simulink model "sovai"  (Simulink 7.5)
settings: Solver=ode45  StartTime=0.0  StopTime=150  FixedStep=1e-2  RelTol=1e-1
PostLoadFcn:
  | % Import the data from Excel for a lookup table
  | data = xlsread('MySpreadsheet','Sheet1');
  | % Row indices for lookup table
  | breakpoints1 = data(2:end,1)';
  | % Column indices for lookup table
  | breakpoints2 = data(1,2:end);
  | % Output values for lookup table
  | table_data = data(2:end,2:end);
values from neighbouring files (symbols this model uses):
  aderdin = 0.8    [InitialParameters.m]
  aderest = 0.88    [InitialParameters.m]
  cons120 = 8.79765621    [InitialParameters.m]
  cons60 = 2.81797722    [InitialParameters.m]
  cons80 = 3.91048967    [InitialParameters.m]
  consvmax = 15.01318082    [InitialParameters.m]
  efemb = [1+cos(-pi+pi*tembc/tefmax)]/2    [InitialParameters.m]
  F0 = 96.9    [InitialParameters.m]
  F2 = 0.502    [InitialParameters.m]
  g = 9.81    [InitialParameters.m]
  m = 825    [InitialParameters.m]
  M1 = 4.273    [InitialParameters.m]
  M2 = 2.238    [InitialParameters.m]
  M3 = 1.444    [InitialParameters.m]
  M4 = 1.029    [InitialParameters.m]
  M5 = 0.838    [InitialParameters.m]
  M6 = 0.838    [InitialParameters.m]
  Md = 4.067    [InitialParameters.m]
  Nfr = 0.6*m*g    (= 4855.95)    [InitialParameters.m]
  Ni = 0.94    [InitialParameters.m]
  Nmax = 6500    [InitialParameters.m]
  Nmin = 1500    [InitialParameters.m]
  Pot = [16.4 19.5 21.9 25.7 29.7 32.8 36.0 38.8 41.4 44.1 47.9 51.9 54.7 57.1 59.2 60.9 61.1 60.9 59.8 59.7 59.3]    [InitialParameters.m]
  rd = 0.274    [InitialParameters.m]
  Rot = [1500 1750 2000 2250 2500 2750 3000 3250 3500 3750 4000 4250 4500 4750 5000 5250 5500 5750 6000 6250 6500]    [InitialParameters.m]
  temb = [temb1,temb2]    [InitialParameters.m]
  teta = 0    [InitialParameters.m]
  Tor = [7.83 7.98 7.84 8.18 8.51 8.54 8.59 8.55 8.47 8.42 8.58 8.75 8.71 8.61 8.48 8.31 7.96 7.59 7.14 6.84 6.53]    [InitialParameters.m]
  Vini = 0    [InitialParameters.m]
libraries: simulink x5, dspswit3 x2
settings Model: Creator=Bruno Silva de Lima  LastModifiedBy=user
settings DebuggingCC: StrictBusMsg=Warning

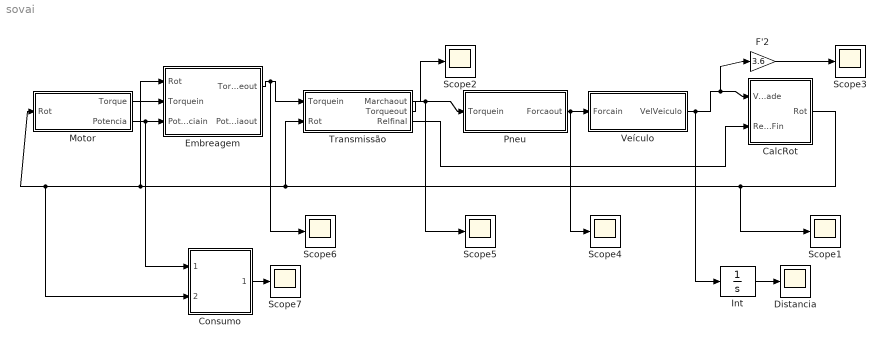
== system sovai ==
  CalcRot : Subsystem
  Consumo : Subsystem
  Distancia : Scope
      settings: SaveName=ScopeData24
  Embreagem : Subsystem  TreatAsAtomicUnit=on
  F'2 : Gain  Gain=3.6  ParameterDataType=fixdt(1, 16)  ParameterScaling=2^0  OutDataType=fixdt(1, 16)  OutScaling=2^0
  Int : Integrator  InitialCondition=Vini
  Motor : Subsystem  TreatAsAtomicUnit=on
  Pneu : Subsystem  TreatAsAtomicUnit=on
  Scope{1..7} (7 alike) : Scope
      Scope1 settings: TimeRange=150  YMin=1500  YMax=6500  MaxDataPoints=200000
      Scope2 settings: SaveName=ScopeData2
      Scope3 settings: TimeRange=0.02579854948784544  YMin=99.96457640249099  YMax=99.99862765668536  SaveName=ScopeData4
      Scope4 settings: SaveName=ScopeData3
      Scope5 settings: SaveName=ScopeData6
      Scope6 settings: SaveName=ScopeData5
      Scope7 settings: SaveName=ScopeData16
  Transmissão : Subsystem  TreatAsAtomicUnit=on
  Veículo : Subsystem  TreatAsAtomicUnit=on
  wires:
  Transmissão/2(Torqueout) -> Pneu/1(Torquein), Scope5/1
  Pneu/1(Forcaout) -> Veículo/1(Forcain), Scope4/1
  Transmissão/3(Relfinal) -> CalcRot/2(RelaçãoFin)
  CalcRot/1(Rot) -> Transmissão/2(Rot), Embreagem/1(Rot), Motor/1(Rot), Consumo/2(rotacao), Scope1/1
  Motor/1(Torque) -> Embreagem/2(Torquein)
  Motor/2(Potencia) -> Embreagem/3(Potênciain), Consumo/1(Potencia)
  Embreagem/1(Torqueout) -> Transmissão/1(Torquein), Scope6/1
  Veículo/1(VelVeiculo) -> CalcRot/1(Velocidade), F'2/1, Int/1
  Transmissão/1(Marchaout) -> Scope2/1
  Consumo/1(consumo) -> Scope7/1
  F'2/1 -> Scope3/1
  Int/1 -> Distancia/1

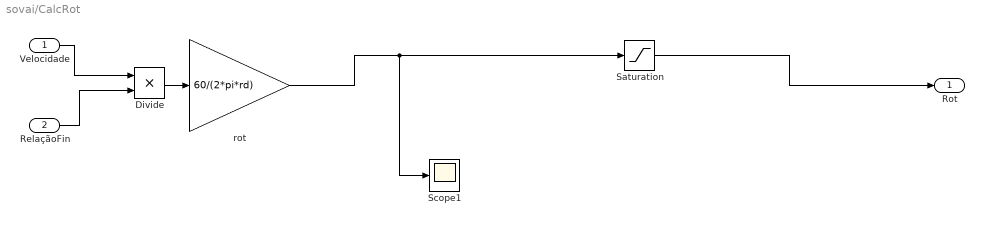
== system sovai/CalcRot ==
  Velocidade : Inport
  RelaçãoFin : Inport  Port=2
  Divide : Product  Inputs=**  OutDataType=fixdt(1, 16)  OutScaling=2^-10
  Saturation : Saturate  UpperLimit=Nmax  LowerLimit=Nmin  OutDataType=fixdt(1, 16)  OutScaling=2^0
  Scope1 : Scope
      settings: SaveName=ScopeData12
  rot : Gain  Gain=60/(2*pi*rd)  ParameterDataType=fixdt(1, 16)  ParameterScaling=2^0  OutDataType=fixdt(1, 16)  OutScaling=2^0
  Rot : Outport
  wires:
  RelaçãoFin/1 -> Divide/2
  Velocidade/1 -> Divide/1
  Divide/1 -> rot/1
  rot/1 -> Scope1/1, Saturation/1
  Saturation/1 -> Rot/1

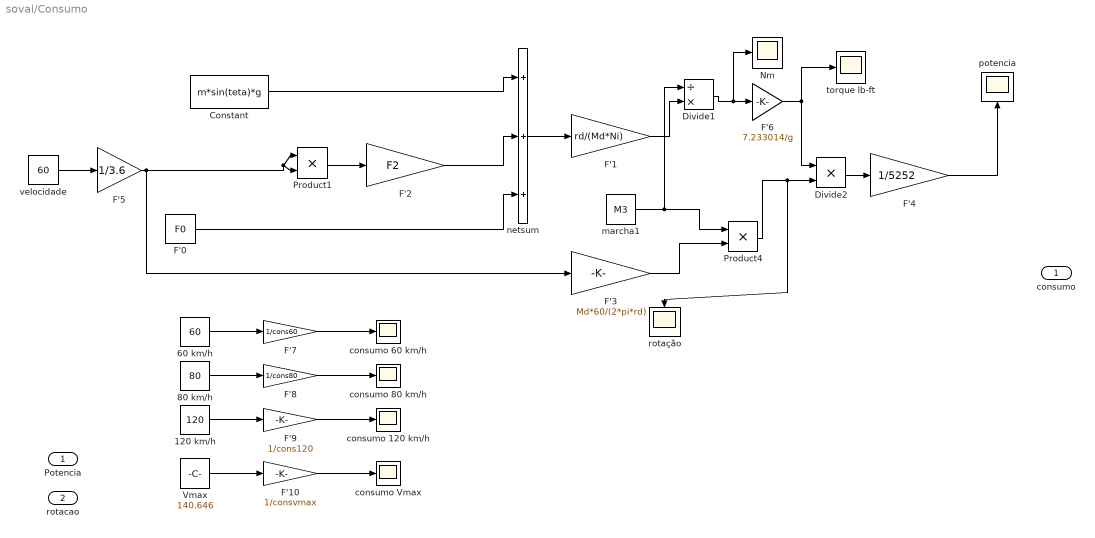
== system sovai/Consumo ==
  Potencia : Inport
  rotacao : Inport  Port=2
  120 km/h : Constant  Value=120  OutDataType=fixdt(1, 16)  OutScaling=2^0
  60 km/h : Constant  Value=60  OutDataType=fixdt(1, 16)  OutScaling=2^0
  80 km/h : Constant  Value=80  OutDataType=fixdt(1, 16)  OutScaling=2^0
  Constant : Constant  Value=m*sin(teta)*g  OutDataType=fixdt(1, 16)  OutScaling=2^0
  Divide1 : Product  Inputs=/*  OutDataType=fixdt(1, 16)  OutScaling=2^-10
  Divide2 : Product  Inputs=**  OutDataType=fixdt(1, 16)  OutScaling=2^-10
  F'0 : Constant  Value=F0  OutDataType=fixdt(1, 16)  OutScaling=2^0
  F'1 : Gain  Gain=rd/(Md*Ni)  ParameterDataType=fixdt(1, 16)  ParameterScaling=2^0  OutDataType=fixdt(1, 16)  OutScaling=2^0
  F'10 : Gain  Gain=1/consvmax  ParameterDataType=fixdt(1, 16)  ParameterScaling=2^0  OutDataType=fixdt(1, 16)  OutScaling=2^0
  F'2 : Gain  Gain=F2  ParameterDataType=fixdt(1, 16)  ParameterScaling=2^0  OutDataType=fixdt(1, 16)  OutScaling=2^0
  F'3 : Gain  Gain=Md*60/(2*pi*rd)  ParameterDataType=fixdt(1, 16)  ParameterScaling=2^0  OutDataType=fixdt(1, 16)  OutScaling=2^0
  F'4 : Gain  Gain=1/5252  ParameterDataType=fixdt(1, 16)  ParameterScaling=2^0  OutDataType=fixdt(1, 16)  OutScaling=2^0
  F'5 : Gain  Gain=1/3.6  ParameterDataType=fixdt(1, 16)  ParameterScaling=2^0  OutDataType=fixdt(1, 16)  OutScaling=2^0
  F'6 : Gain  Gain=7.233014/g  ParameterDataType=fixdt(1, 16)  ParameterScaling=2^0  OutDataType=fixdt(1, 16)  OutScaling=2^0
  F'7 : Gain  Gain=1/cons60  ParameterDataType=fixdt(1, 16)  ParameterScaling=2^0  OutDataType=fixdt(1, 16)  OutScaling=2^0
  F'8 : Gain  Gain=1/cons80  ParameterDataType=fixdt(1, 16)  ParameterScaling=2^0  OutDataType=fixdt(1, 16)  OutScaling=2^0
  F'9 : Gain  Gain=1/cons120  ParameterDataType=fixdt(1, 16)  ParameterScaling=2^0  OutDataType=fixdt(1, 16)  OutScaling=2^0
  Nm : Scope
      settings: SaveName=ScopeData20
  Product1 : Product  OutDataType=fixdt(1, 16)  OutScaling=2^0  RndMeth=Zero
  Product4 : Product  OutDataType=fixdt(1, 16)  OutScaling=2^0  RndMeth=Zero
  Vmax : Constant  Value=140.646  OutDataType=fixdt(1, 16)  OutScaling=2^0
  consumo 120 km/h : Scope
      settings: SaveName=ScopeData22
  consumo 60 km/h : Scope
  consumo 80 km/h : Scope
      settings: SaveName=ScopeData21
  consumo Vmax : Scope
      settings: SaveName=ScopeData23
  marcha1 : Constant  Value=M3  OutDataType=fixdt(1, 16)  OutScaling=2^0
  netsum : Sum  Inputs=+++  OutDataType=sfix(16)  OutScaling=2^0  SaturateOnIntegerOverflow=on  InputSameDT=on  OutDataTypeStr=Inherit: Same as first input
  potencia : Scope
      settings: SaveName=ScopeData18
  rotação : Scope
      settings: SaveName=ScopeData17
  torque lb-ft : Scope
      settings: SaveName=ScopeData19
  velocidade : Constant  Value=60  OutDataType=fixdt(1, 16)  OutScaling=2^0
  consumo : Outport
  wires:
  Constant/1 -> netsum/1
  F'2/1 -> netsum/2
  Product1/1 -> F'2/1
  F'0/1 -> netsum/3
  velocidade/1 -> F'5/1
  netsum/1 -> F'1/1
  F'1/1 -> Divide1/2
  F'3/1 -> Product4/2
  marcha1/1 -> Product4/1, Divide1/1
  Product4/1 -> rotação/1, Divide2/2
  Divide1/1 -> F'6/1, Nm/1
  Divide2/1 -> F'4/1
  F'4/1 -> potencia/1
  F'5/1 -> Product1/1, Product1/2, F'3/1
  F'6/1 -> Divide2/1, torque lb-ft/1
  60 km/h/1 -> F'7/1
  80 km/h/1 -> F'8/1
  120 km/h/1 -> F'9/1
  Vmax/1 -> F'10/1
  F'9/1 -> consumo 120 km/h/1
  F'8/1 -> consumo 80 km/h/1
  F'7/1 -> consumo 60 km/h/1
  F'10/1 -> consumo Vmax/1

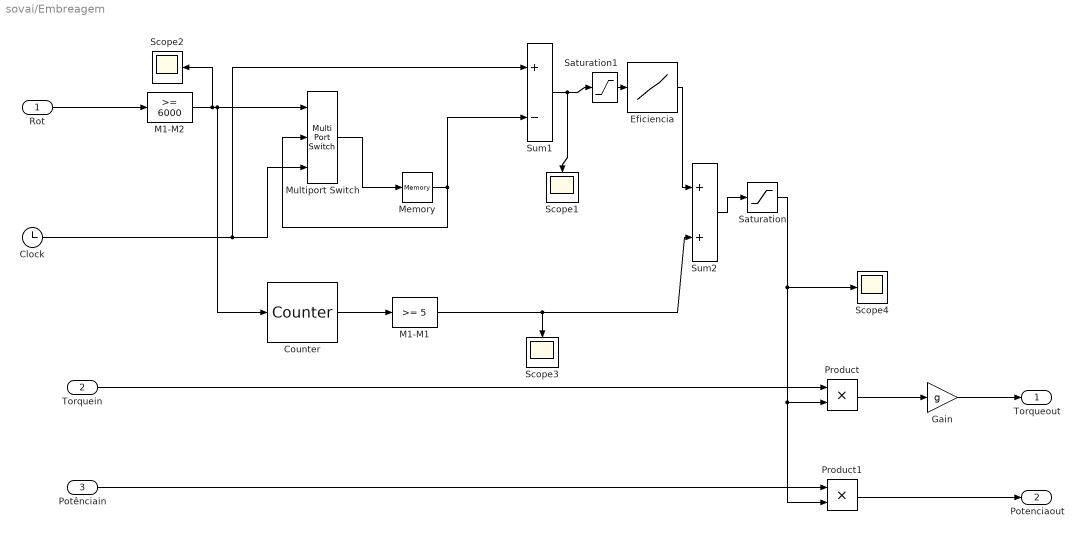
== system sovai/Embreagem ==
  Rot : Inport  OutDataType=fixdt(1, 16)  OutScaling=2^0
  Torquein : Inport  Port=2  OutDataType=fixdt(1, 16)  OutScaling=2^0
  Potênciain : Inport  Port=3  OutDataType=fixdt(1, 16)  OutScaling=2^0
  Clock : Clock
      settings: Decimation=10
  Counter : dspswit3/Counter  Direction=Up  CountEvent=Rising edge  CounterSize=User defined  MaxCount=6  InitialCount=1  Output=Count  HitValue=32  ResetInput=off  SamplesPerFrame=1  Ts=1  CntDtype=double  HitDtype=Logical
  Eficiencia : Lookup  InputValues=temb  Table=efemb  OutDataType=fixdt(1, 16)  OutScaling=2^0
  Gain : Gain  Gain=g  ParameterDataType=fixdt(1, 16)  ParameterScaling=2^0  OutDataType=fixdt(1, 16)  OutScaling=2^0
  M1-M1 : simulink/Logic and Bit Operations/Compare To Constant  SystemSampleTime=-1  relop=>=  const=5  LogicOutDataTypeMode=uint8
  M1-M2 : simulink/Logic and Bit Operations/Compare To Constant  SystemSampleTime=-1  relop=>=  const=6000  LogicOutDataTypeMode=uint8
  Memory : Memory
  Multiport Switch : MultiPortSwitch  DataPortOrder=Zero-based contiguous  Inputs=2  zeroidx=on  OutDataType=fixdt(1, 16)  OutScaling=2^0
  Product : Product  OutDataType=fixdt(1, 16)  OutScaling=2^0  RndMeth=Zero
  Product1 : Product  OutDataType=fixdt(1, 16)  OutScaling=2^0  RndMeth=Zero
  Saturation : Saturate  UpperLimit=1  LowerLimit=0  OutDataType=fixdt(1, 16)  OutScaling=2^0
  Saturation1 : Saturate  UpperLimit=1.5  LowerLimit=0  OutDataType=fixdt(1, 16)  OutScaling=2^0
  Scope{1..4} (4 alike) : Scope
      Scope1 settings: SaveName=ScopeData13
      Scope2 settings: SaveName=ScopeData14
      Scope3 settings: SaveName=ScopeData9
      Scope4 settings: SaveName=ScopeData25
  Sum1 : Sum  Inputs=+-  OutDataType=fixdt(1, 16)  OutScaling=2^0
  Sum2 : Sum  Inputs=2  OutDataType=fixdt(1, 16)  OutScaling=2^0
  Torqueout : Outport  OutDataType=fixdt(1, 16)  OutScaling=2^0
  Potenciaout : Outport  Port=2  OutDataType=fixdt(1, 16)  OutScaling=2^0
  wires:
  Product/1 -> Gain/1
  Product1/1 -> Potenciaout/1
  Torquein/1 -> Product/1
  Potênciain/1 -> Product1/1
  Rot/1 -> M1-M2/1
  Saturation/1 -> Product1/2, Product/2, Scope4/1
  Saturation1/1 -> Eficiencia/1
  Multiport Switch/1 -> Memory/1
  Memory/1 -> Sum1/2, Multiport Switch/2
  Clock/1 -> Multiport Switch/3, Sum1/1
  Sum1/1 -> Saturation1/1, Scope1/1
  Gain/1 -> Torqueout/1
  M1-M2/1 -> Scope2/1, Multiport Switch/1, Counter/1
  Counter/1 -> M1-M1/1
  M1-M1/1 -> Sum2/2, Scope3/1
  Sum2/1 -> Saturation/1
  Eficiencia/1 -> Sum2/1

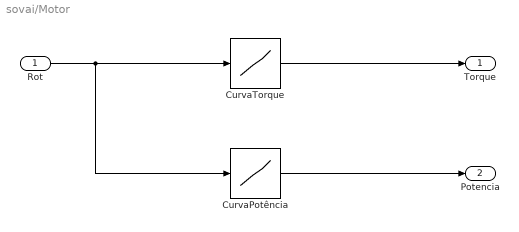
== system sovai/Motor ==
  Rot : Inport  OutDataType=fixdt(1, 16)  OutScaling=2^0
  CurvaPotência : Lookup  InputValues=Rot  Table=Pot  OutDataType=fixdt(1, 16)  OutScaling=2^0
  CurvaTorque : Lookup  InputValues=Rot  Table=Tor  OutDataType=fixdt(1, 16)  OutScaling=2^0
  Torque : Outport  OutDataType=fixdt(1, 16)  OutScaling=2^0
  Potencia : Outport  Port=2  OutDataType=fixdt(1, 16)  OutScaling=2^0
  wires:
  CurvaTorque/1 -> Torque/1
  CurvaPotência/1 -> Potencia/1
  Rot/1 -> CurvaTorque/1, CurvaPotência/1

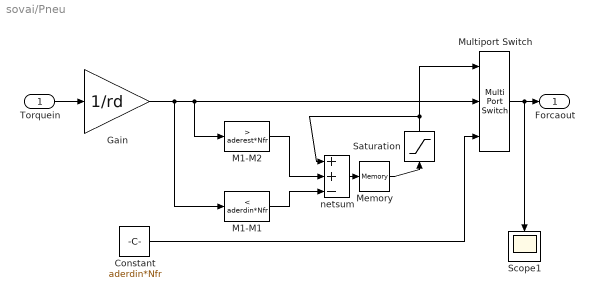
== system sovai/Pneu ==
  Torquein : Inport  OutDataType=fixdt(1, 16)  OutScaling=2^0
  Constant : Constant  Value=aderdin*Nfr  OutDataType=fixdt(1, 16)  OutScaling=2^0
  Gain : Gain  Gain=1/rd  ParameterDataType=fixdt(1, 16)  ParameterScaling=2^0  OutDataType=fixdt(1, 16)  OutScaling=2^0
  M1-M1 : simulink/Logic and Bit Operations/Compare To Constant  SystemSampleTime=-1  relop=<  const=aderdin*Nfr  LogicOutDataTypeMode=uint8
  M1-M2 : simulink/Logic and Bit Operations/Compare To Constant  SystemSampleTime=-1  relop=>  const=aderest*Nfr  LogicOutDataTypeMode=uint8
  Memory : Memory
  Multiport Switch : MultiPortSwitch  DataPortOrder=Zero-based contiguous  Inputs=2  zeroidx=on  OutDataType=fixdt(1, 16)  OutScaling=2^0
  Saturation : Saturate  UpperLimit=1  LowerLimit=0  OutDataType=fixdt(1, 16)  OutScaling=2^0
  Scope1 : Scope
      settings: SaveName=ScopeData26  MaxDataPoints=200000
  netsum : Sum  Inputs=++-  OutDataType=sfix(16)  OutScaling=2^0  SaturateOnIntegerOverflow=on  InputSameDT=on  OutDataTypeStr=Inherit: Same as first input
  Forcaout : Outport  OutDataType=fixdt(1, 16)  OutScaling=2^0
  wires:
  Torquein/1 -> Gain/1
  Multiport Switch/1 -> Forcaout/1, Scope1/1
  Constant/1 -> Multiport Switch/3
  Memory/1 -> Saturation/1
  M1-M2/1 -> netsum/2
  M1-M1/1 -> netsum/3
  netsum/1 -> Memory/1
  Saturation/1 -> Multiport Switch/1, netsum/1
  Gain/1 -> Multiport Switch/2, M1-M2/1, M1-M1/1

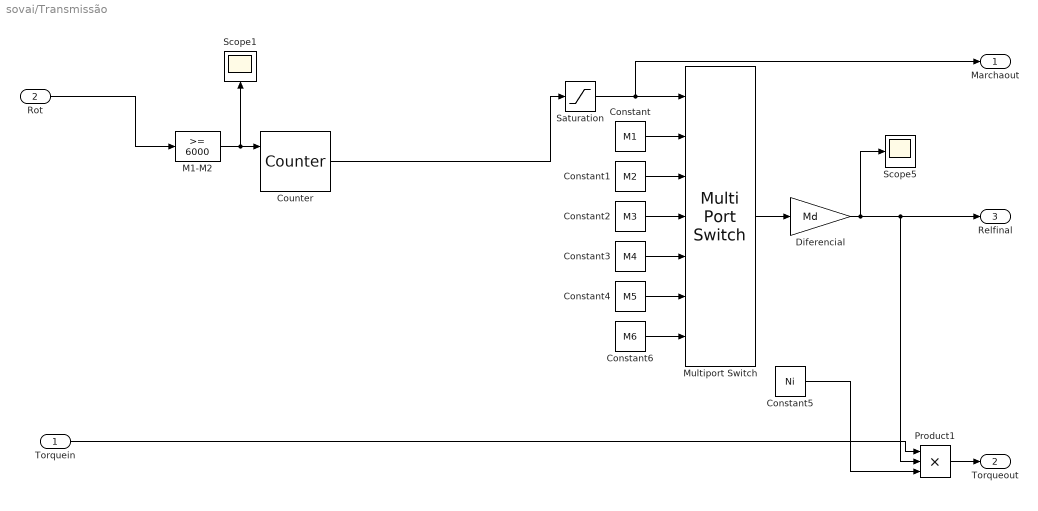
== system sovai/Transmissão ==
  Torquein : Inport  OutDataType=fixdt(1, 16)  OutScaling=2^0
  Rot : Inport  Port=2  OutDataType=fixdt(1, 16)  OutScaling=2^0
  Constant : Constant  Value=M1  OutDataType=fixdt(1, 16)  OutScaling=2^0
  Constant1 : Constant  Value=M2  OutDataType=fixdt(1, 16)  OutScaling=2^0
  Constant2 : Constant  Value=M3  OutDataType=fixdt(1, 16)  OutScaling=2^0
  Constant3 : Constant  Value=M4  OutDataType=fixdt(1, 16)  OutScaling=2^0
  Constant4 : Constant  Value=M5  OutDataType=fixdt(1, 16)  OutScaling=2^0
  Constant5 : Constant  Value=Ni  OutDataType=fixdt(1, 16)  OutScaling=2^0
  Constant6 : Constant  Value=M6  OutDataType=fixdt(1, 16)  OutScaling=2^0
  Counter : dspswit3/Counter  Direction=Up  CountEvent=Rising edge  CounterSize=User defined  MaxCount=6  InitialCount=1  Output=Count  HitValue=32  ResetInput=on  SamplesPerFrame=1  Ts=1  CntDtype=double  HitDtype=Logical
  Diferencial : Gain  Gain=Md  ParameterDataType=fixdt(1, 16)  ParameterScaling=2^0  OutDataType=fixdt(1, 16)  OutScaling=2^0
  M1-M2 : simulink/Logic and Bit Operations/Compare To Constant  SystemSampleTime=-1  relop=>=  const=6000  LogicOutDataTypeMode=uint8
  Multiport Switch : MultiPortSwitch  Inputs=6  zeroidx=off  OutDataType=fixdt(1, 16)  OutScaling=2^0
  Product1 : Product  Inputs=3  OutDataType=fixdt(1, 16)  OutScaling=2^0  RndMeth=Zero
  Saturation : Saturate  UpperLimit=4  LowerLimit=1  OutDataType=fixdt(1, 16)  OutScaling=2^0
  Scope1 : Scope
      settings: SaveName=ScopeData15
  Scope5 : Scope
      settings: SaveName=ScopeData11
  Marchaout : Outport  OutDataType=fixdt(1, 16)  OutScaling=2^0
  Torqueout : Outport  Port=2  OutDataType=fixdt(1, 16)  OutScaling=2^0
  Relfinal : Outport  Port=3  OutDataType=fixdt(1, 16)  OutScaling=2^0
  wires:
  Constant/1 -> Multiport Switch/2
  Constant1/1 -> Multiport Switch/3
  Constant2/1 -> Multiport Switch/4
  Constant3/1 -> Multiport Switch/5
  Constant4/1 -> Multiport Switch/6
  Constant6/1 -> Multiport Switch/7
  Product1/1 -> Torqueout/1
  Torquein/1 -> Product1/1
  Diferencial/1 -> Scope5/1, Product1/2, Relfinal/1
  Saturation/1 -> Multiport Switch/1, Marchaout/1
  Constant5/1 -> Product1/3
  Rot/1 -> M1-M2/1
  M1-M2/1 -> Counter/1, Scope1/1
  Counter/1 -> Saturation/1
  Multiport Switch/1 -> Diferencial/1

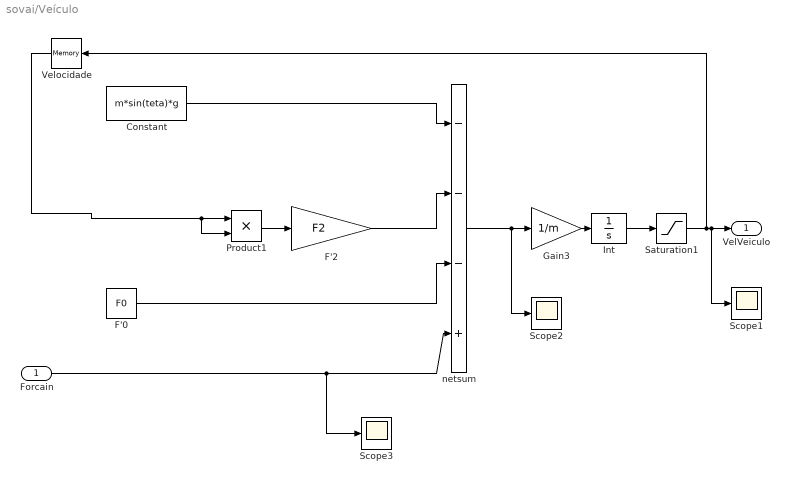
== system sovai/Veículo ==
  Forcain : Inport  OutDataType=fixdt(1, 16)  OutScaling=2^0
  Constant : Constant  Value=m*sin(teta)*g  OutDataType=fixdt(1, 16)  OutScaling=2^0
  F'0 : Constant  Value=F0  OutDataType=fixdt(1, 16)  OutScaling=2^0
  F'2 : Gain  Gain=F2  ParameterDataType=fixdt(1, 16)  ParameterScaling=2^0  OutDataType=fixdt(1, 16)  OutScaling=2^0
  Gain3 : Gain  Gain=1/m  ParameterDataType=fixdt(1, 16)  ParameterScaling=2^0  OutDataType=fixdt(1, 16)  OutScaling=2^0
  Int : Integrator  InitialCondition=Vini
  Product1 : Product  OutDataType=fixdt(1, 16)  OutScaling=2^0  RndMeth=Zero
  Saturation1 : Saturate  UpperLimit=9999  LowerLimit=0  OutDataType=fixdt(1, 16)  OutScaling=2^0
  Scope1 : Scope
      settings: SaveName=ScopeData7
  Scope2 : Scope
      settings: SaveName=ScopeData8
  Scope3 : Scope
      settings: SaveName=ScopeData10
  Velocidade : Memory  X0=Vini
  netsum : Sum  Inputs=---+  OutDataType=sfix(16)  OutScaling=2^0  SaturateOnIntegerOverflow=on  InputSameDT=on  OutDataTypeStr=Inherit: Same as first input
  VelVeiculo : Outport  OutDataType=fixdt(1, 16)  OutScaling=2^0
  wires:
  Constant/1 -> netsum/1
  Velocidade/1 -> Product1/1, Product1/2
  Gain3/1 -> Int/1
  netsum/1 -> Gain3/1, Scope2/1
  Forcain/1 -> netsum/4, Scope3/1
  Int/1 -> Saturation1/1
  F'2/1 -> netsum/2
  Product1/1 -> F'2/1
  F'0/1 -> netsum/3
  Saturation1/1 -> Velocidade/1, VelVeiculo/1, Scope1/1
